simulink model "MPC_variants_20"  (R2026a)
settings: Solver=FixedStepAuto
settings Model: Creator=rayyu  LastModifiedBy=rayyu
settings RTWCC: SystemTargetFile=ert.tlc  Description=Embedded Coder
settings ERTTargetCC: GenerateSampleERTMain=on

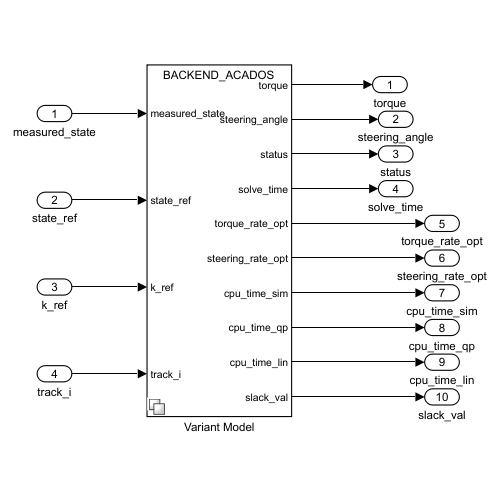
[thumbnail: Simulink's stored preview of the top-level diagram]
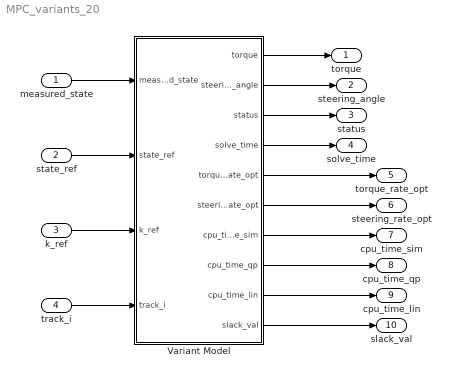
== system MPC_variants_20 ==
  measured_state : Inport
  state_ref : Inport  Port=2
  k_ref : Inport  Port=3
  track_i : Inport  Port=4
  Variant Model : Subsystem  Variant=on
  torque : Outport
  steering_angle : Outport  Port=2
  status : Outport  Port=3
  solve_time : Outport  Port=4
  torque_rate_opt : Outport  Port=5
  steering_rate_opt : Outport  Port=6
  cpu_time_sim : Outport  Port=7
  cpu_time_qp : Outport  Port=8
  cpu_time_lin : Outport  Port=9
  slack_val : Outport  Port=10
  wires:
  measured_state/1 -> Variant Model/1(measured_state)
  state_ref/1 -> Variant Model/2(state_ref)
  k_ref/1 -> Variant Model/3(k_ref)
  track_i/1 -> Variant Model/4(track_i)
  Variant Model/1(torque) -> torque/1
  Variant Model/2(steering_angle) -> steering_angle/1
  Variant Model/3(status) -> status/1
  Variant Model/4(solve_time) -> solve_time/1
  Variant Model/8(cpu_time_qp) -> cpu_time_qp/1
  Variant Model/6(steering_rate_opt) -> steering_rate_opt/1
  Variant Model/9(cpu_time_lin) -> cpu_time_lin/1
  Variant Model/10(slack_val) -> slack_val/1
  Variant Model/7(cpu_time_sim) -> cpu_time_sim/1
  Variant Model/5(torque_rate_opt) -> torque_rate_opt/1

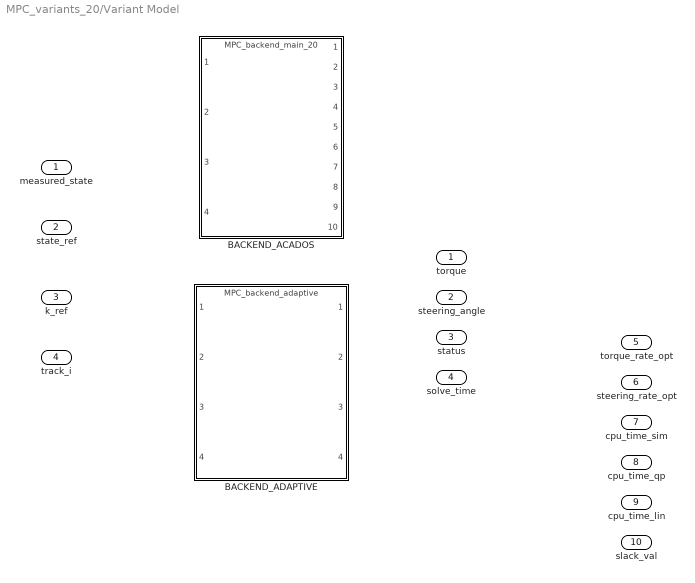
== system MPC_variants_20/Variant Model ==
  measured_state : Inport
  state_ref : Inport  Port=2
  k_ref : Inport  Port=3
  track_i : Inport  Port=4
  BACKEND_ACADOS : ModelReference  ModelNameDialog=MPC_backend_main_20.slx  SimulationMode=Normal  VariantControl=controllerParams.controller_backend == 1  ModelReferenceVersion=1.105
  BACKEND_ADAPTIVE : ModelReference  ModelNameDialog=MPC_backend_adaptive.slx  SimulationMode=Normal  VariantControl=controllerParams.controller_backend == 2  ModelReferenceVersion=1.48
  torque : Outport
  steering_angle : Outport  Port=2
  status : Outport  Port=3
  solve_time : Outport  Port=4
  torque_rate_opt : Outport  Port=5
  steering_rate_opt : Outport  Port=6
  cpu_time_sim : Outport  Port=7
  cpu_time_qp : Outport  Port=8
  cpu_time_lin : Outport  Port=9
  slack_val : Outport  Port=10
